simulink model "BBBC"  (R2022b)
settings: Solver=VariableStepAuto  StartTime=0.0  StopTime=0.5  RelTol=1e-3
undefined symbols (not defined in the file): dct, dEv, Ev, sigbuilder_block
libraries: spsSeriesRLCBranchLib x5, spsMosfetLib x4, simulink x3, spsVoltageMeasurementLib x2, spsGroundLib x1, spsCurrentMeasurementLib x1, spsControlledVoltageSourceLib x1, spspowerguiLib x1
settings Model: Creator=Dopechuro  LastModifiedBy=Dopechuro

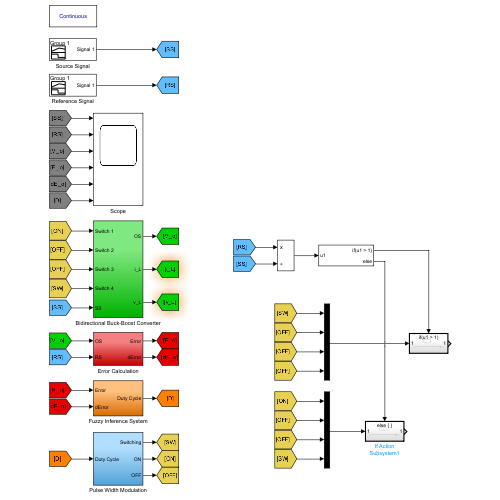
[thumbnail: Simulink's stored preview of the top-level diagram]
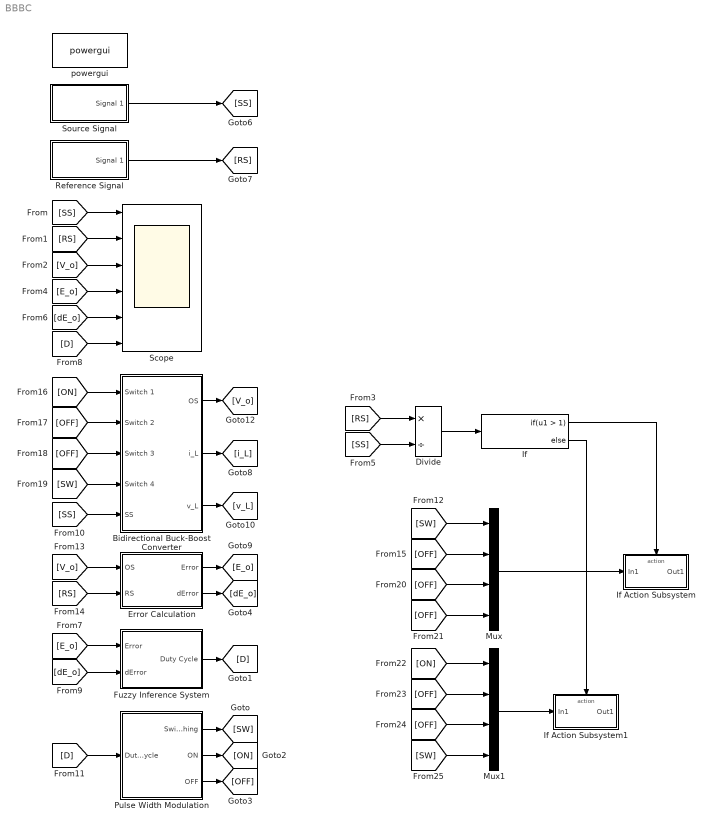
== system BBBC ==
  Bidirectional Buck-Boost Converter : Subsystem
  Divide : Product  Inputs=*/
  Error Calculation : Subsystem
  Fuzzy Inference System : Subsystem
  If : If  IfExpression=u1 > 1
  If Action Subsystem : Subsystem  TreatAsAtomicUnit=on
  If Action Subsystem1 : Subsystem  TreatAsAtomicUnit=on
  Mux : Mux
  Mux1 : Mux
  Pulse Width Modulation : Subsystem
  Reference Signal : Subsystem  Tag=STV Subsys  LoadFcn=sigbuilder_block('load');  StartFcn=sigbuilder_block('start');  StopFcn=sigbuilder_block('stop');  ClipboardFcn=sigbuilder_block('clipboard');  mask(Sigbuilder block){tuvar=[0:10]}
      mask help: Simulink:masks:SigbuilderBlock_MD
      mask init:
      | if ~strcmp(get_param(bdroot(gcbh),'SimulationStatus'),'stopped') tuvar = sigbuilder_block('maskInit'); end
      settings: CopyFcn=sigbuilder_block('copy');  DeleteFcn=sigbuilder_block('delete');  ModelCloseFcn=sigbuilder_block('modelClose');  PreSaveFcn=sigbuilder_block('preSave');  PauseFcn=sigbuilder_block('pause');  ContinueFcn=sigbuilder_block('continue');  NameChangeFcn=sigbuilder_block('namechange');  OpenFcn=sigbuilder_block('open',[530.25 309.75 550.5 399.75 ]);  CloseFcn=sigbuilder_block('close');
      mask Display: plot(0, 0, 100, 100,[2, 2, 32, 32, 2], [68, 8, 8, 68, 68],[32, 2], [38, 38], [32, 19, 2],[53, 60, 44], [32, 17, 17, 2],[16, 16, 31, 31]);txt = getActiveGroup(gcbh);text(2, 100, txt,'verticalAlignment', 'top');
  Scope : Scope  NumInputPorts=6
  Source Signal : Subsystem  Tag=STV Subsys  LoadFcn=sigbuilder_block('load');  StartFcn=sigbuilder_block('start');  StopFcn=sigbuilder_block('stop');  ClipboardFcn=sigbuilder_block('clipboard');  mask(Sigbuilder block){tuvar=[0:10]}
      mask help: Simulink:masks:SigbuilderBlock_MD
      mask init:
      | if ~strcmp(get_param(bdroot(gcbh),'SimulationStatus'),'stopped') tuvar = sigbuilder_block('maskInit'); end
      settings: CopyFcn=sigbuilder_block('copy');  DeleteFcn=sigbuilder_block('delete');  ModelCloseFcn=sigbuilder_block('modelClose');  PreSaveFcn=sigbuilder_block('preSave');  PauseFcn=sigbuilder_block('pause');  ContinueFcn=sigbuilder_block('continue');  NameChangeFcn=sigbuilder_block('namechange');  OpenFcn=sigbuilder_block('open',[395.25 256.5 550.5 399.75 ]);  CloseFcn=sigbuilder_block('close');
      mask Display: plot(0, 0, 100, 100,[2, 2, 32, 32, 2], [68, 8, 8, 68, 68],[32, 2], [38, 38], [32, 19, 2],[53, 60, 44], [32, 17, 17, 2],[16, 16, 31, 31]);txt = getActiveGroup(gcbh);text(2, 100, txt,'verticalAlignment', 'top');
  powergui : spspowerguiLib/powergui  Priority=1  SimulationMode=Continuous  SampleTime=50e-6  frequency=60  Iterations=50  frequencyindice=0  Pbase=100e6  ErrMax=1e-4  UnitsV=kV  UnitsW=MW  buscounter=0  FunctionMessages=off  echomessages=off  EnableUseOfTLC=off  CurrentSourceSwitches=off  DisableSnubberDevices=off  DisableRonSwitches=off  DisableVfSwitches=off  DisplayEquations=off  AutomaticDiscreteSolvers=off  SolverType=Tustin/Backward Euler (TBE)  Interpol=off  ExternalGateDelay=off  methode=off  Ts=100  x0status=blocks  SPID=on  SwTol=0  HookPort=off  NonlinearTolerance=1e-4  nMaxIteration=100  ContinueOnMaxIteration=off  RestoreLinks=warning  ResistiveCurrentMeasurement=off  Frange=[0:2:500]  Ylog=off  Xlog=on  ShowGrid=off  save=off  variable=ZData  structure=0  ZoomFFT=off  StartTime=0.0  cycles=1  DisplayStyle=1  fundamental=60  FreqAxis=off  MaxFrequency=1000  frequencyindicesteady=1  RmsSteady=1  display=off
  wires:
  [RS] -> Scope/2
  [V_o] -> Scope/3
  [E_o] -> Scope/4
  [dE_o] -> Scope/5
  [D] -> Scope/6
  Source Signal/1(Signal 1) -> [SS]
  Reference Signal/1(Signal 1) -> [RS]
  [V_o] -> Error Calculation/1(OS)
  [RS] -> Error Calculation/2(RS)
  Error Calculation/1(Error) -> [E_o]
  Error Calculation/2(dError) -> [dE_o]
  [SS] -> Scope/1
  [ON] -> Bidirectional Buck-Boost Converter/1(Switch 1)
  [OFF] -> Bidirectional Buck-Boost Converter/2(Switch 2)
  [OFF] -> Bidirectional Buck-Boost Converter/3(Switch 3)
  [SW] -> Bidirectional Buck-Boost Converter/4(Switch 4)
  [SS] -> Bidirectional Buck-Boost Converter/5(SS)
  Bidirectional Buck-Boost Converter/1(OS) -> [V_o]
  Bidirectional Buck-Boost Converter/2(i_L) -> [i_L]
  Bidirectional Buck-Boost Converter/3(v_L) -> [v_L]
  [E_o] -> Fuzzy Inference System/1(Error)
  [dE_o] -> Fuzzy Inference System/2(dError)
  Fuzzy Inference System/1(Duty Cycle) -> [D]
  [D] -> Pulse Width Modulation/1(Duty Cycle)
  Pulse Width Modulation/1(Switching) -> [SW]
  Pulse Width Modulation/2(ON) -> [ON]
  Pulse Width Modulation/3(OFF) -> [OFF]
  [SS] -> Divide/2
  [RS] -> Divide/1
  [SW] -> Mux/1
  [OFF] -> Mux/2
  [OFF] -> Mux/3
  [OFF] -> Mux/4
  [ON] -> Mux1/1
  [OFF] -> Mux1/2
  [OFF] -> Mux1/3
  [SW] -> Mux1/4
  Divide/1 -> If/1
  If/1 -> If Action Subsystem/Action
  If/2 -> If Action Subsystem1/Action
  Mux1/1 -> If Action Subsystem1/1(In1)
  Mux/1 -> If Action Subsystem/1(In1)

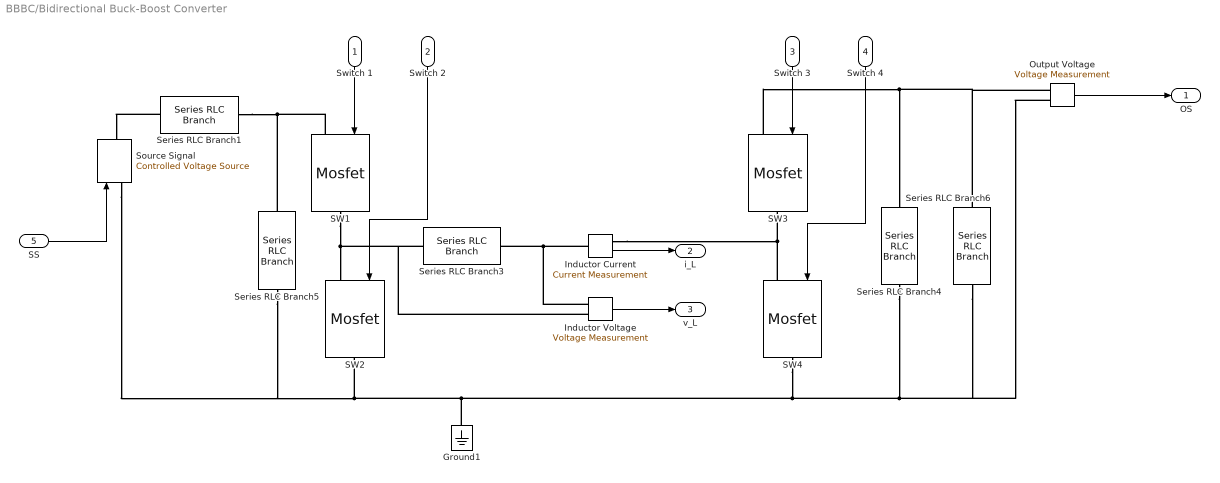
== system BBBC/Bidirectional Buck-Boost Converter ==
  Switch 1 : Inport
  Switch 2 : Inport  Port=2
  Switch 3 : Inport  Port=3
  Switch 4 : Inport  Port=4
  SS : Inport  Port=5
  Ground1 : spsGroundLib/Ground  LConnTagsString=a
  Inductor Current : spsCurrentMeasurementLib/Current Measurement  PhasorSimulation=off  OutputType=Complex  PSBequivalent=0
  Inductor Voltage : spsVoltageMeasurementLib/Voltage Measurement  PhasorSimulation=off  OutputType=Complex  PSBequivalent=0
  Output Voltage : spsVoltageMeasurementLib/Voltage Measurement  PhasorSimulation=off  OutputType=Complex  PSBequivalent=0
  SW{1..4} (4 alike) : spsMosfetLib/Mosfet  Ron=0.1  Lon=0  Rd=0.01  Vfd=0  IC=0  Rs=1e5  Cs=inf  Measurements=off
  Series RLC Branch1 : spsSeriesRLCBranchLib/Series RLC Branch  LConnTagsString=__new0  RConnTagsString=__new0  BranchType=R  Resistance=1e-6  Inductance=1e-3  SetiL0=off  InitialCurrent=0  Capacitance=1e-6  Setx0=off  InitialVoltage=0  Measurements=None
  Series RLC Branch3 : spsSeriesRLCBranchLib/Series RLC Branch  LConnTagsString=__new0  RConnTagsString=__new0  BranchType=L  Resistance=1  Inductance=22e-6  SetiL0=off  InitialCurrent=0  Capacitance=1e-6  Setx0=off  InitialVoltage=0  Measurements=None
  Series RLC Branch4 : spsSeriesRLCBranchLib/Series RLC Branch  LConnTagsString=__new0  RConnTagsString=__new0  BranchType=C  Resistance=1  Inductance=1e-3  SetiL0=off  InitialCurrent=0  Capacitance=1000e-6  Setx0=off  InitialVoltage=0  Measurements=None
  Series RLC Branch5 : spsSeriesRLCBranchLib/Series RLC Branch  LConnTagsString=__new0  RConnTagsString=__new0  BranchType=C  Resistance=1  Inductance=1e-3  SetiL0=off  InitialCurrent=0  Capacitance=1000e-6  Setx0=off  InitialVoltage=0  Measurements=None
  Series RLC Branch6 : spsSeriesRLCBranchLib/Series RLC Branch  LConnTagsString=__new0  RConnTagsString=__new0  BranchType=R  Resistance=5  Inductance=1e-3  SetiL0=off  InitialCurrent=0  Capacitance=1e-6  Setx0=off  InitialVoltage=0  Measurements=None
  Source Signal : spsControlledVoltageSourceLib/Controlled Voltage Source  Initialize=off  Source_Type=DC  Amplitude=0  Phase=0  Frequency=0  Measurements=None
  OS : Outport
  i_L : Outport  Port=2
  v_L : Outport  Port=3
  wires:
  Switch 1/1 -> SW1/1
  Switch 3/1 -> SW3/1
  Switch 2/1 -> SW2/1
  SS/1 -> Source Signal/1
  Switch 4/1 -> SW4/1
  Inductor Current/1 -> i_L/1
  Output Voltage/1 -> OS/1
  Inductor Voltage/1 -> v_L/1
  connections:
  Series RLC Branch5/LConn1 -- Series RLC Branch1/RConn1 -- SW1/LConn1
  Inductor Current/LConn1 -- Inductor Voltage/LConn2 -- Series RLC Branch3/RConn1
  SW4/LConn1 -- Inductor Current/RConn1 -- SW3/RConn1
  SW4/RConn1 -- Series RLC Branch6/RConn1 -- Output Voltage/LConn2 -- Series RLC Branch4/RConn1 -- Ground1/LConn1 -- Source Signal/LConn1 -- Series RLC Branch5/RConn1 -- SW2/RConn1
  SW1/RConn1 -- Inductor Voltage/LConn1 -- Series RLC Branch3/LConn1 -- SW2/LConn1
  Series RLC Branch1/LConn1 -- Source Signal/RConn1
  SW3/LConn1 -- Output Voltage/LConn1 -- Series RLC Branch6/LConn1 -- Series RLC Branch4/LConn1

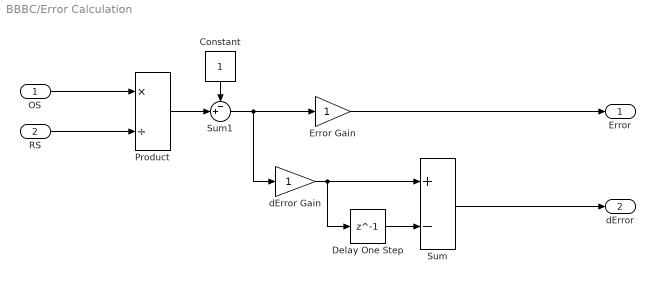
== system BBBC/Error Calculation ==
  OS : Inport
  RS : Inport  Port=2
  Constant : Constant
  Delay One Step : Delay  DelayLength=1
  Error Gain : Gain
  Product : Product  Inputs=*/
  Sum : Sum  Inputs=+-
  Sum1 : Sum  Inputs=-+|
  dError Gain : Gain
  Error : Outport
  dError : Outport  Port=2
  wires:
  Sum1/1 -> dError Gain/1, Error Gain/1
  dError Gain/1 -> Sum/1, Delay One Step/1
  Error Gain/1 -> Error/1
  Constant/1 -> Sum1/1
  Delay One Step/1 -> Sum/2
  Product/1 -> Sum1/2
  Sum/1 -> dError/1
  OS/1 -> Product/1
  RS/1 -> Product/2

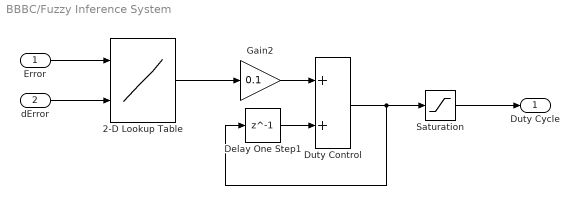
== system BBBC/Fuzzy Inference System ==
  Error : Inport
  dError : Inport  Port=2
  2-D Lookup Table : Lookup_n-D  LookupTableObject=''  BreakpointsForDimension1=Ev  BreakpointsForDimension2=dEv  BreakpointsForDimension1FirstPoint=10  BreakpointsForDimension2FirstPoint=10  BreakpointsForDimension1Spacing=12  BreakpointsForDimension2Spacing=12  IndexSearchMethod=Evenly spaced points  Table=dct  InterpMethod=Nearest  DiagnosticForOutOfRangeInput=Warning  InternalRulePriority=Speed  OutDataTypeStr=Inherit: Inherit from 'Table data'  RndMeth=Simplest
      settings: InputPortMap=u0,u1
  Delay One Step1 : Delay  DelayLength=1
  Duty Control : Sum
  Gain2 : Gain  Gain=0.1
  Saturation : Saturate  UpperLimit=0.4  LowerLimit=-0.4
  Duty Cycle : Outport
  wires:
  Delay One Step1/1 -> Duty Control/2
  Duty Control/1 -> Saturation/1, Delay One Step1/1
  Gain2/1 -> Duty Control/1
  2-D Lookup Table/1 -> Gain2/1
  Saturation/1 -> Duty Cycle/1
  Error/1 -> 2-D Lookup Table/1
  dError/1 -> 2-D Lookup Table/2

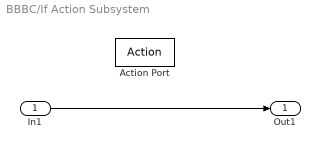
== system BBBC/If Action Subsystem ==
  In1 : Inport
  Action Port : ActionPort  ActionPortLabel=if(u1 > 1)
  Out1 : Outport
  wires:
  In1/1 -> Out1/1

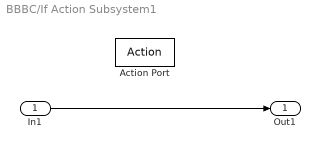
== system BBBC/If Action Subsystem1 ==
  In1 : Inport
  Action Port : ActionPort  ActionPortLabel=else
  Out1 : Outport
  wires:
  In1/1 -> Out1/1

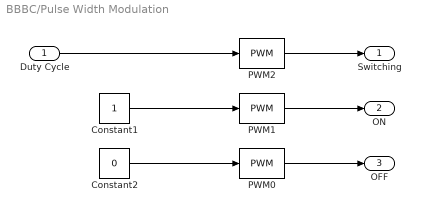
== system BBBC/Pulse Width Modulation ==
  Duty Cycle : Inport
  Constant1 : Constant
  Constant2 : Constant  Value=0
  PWM0 : simulink/Discontinuities/PWM  DisableCoverage=on  Period=1/1e4  InitialDelay=0  DisallowZeroDutyCycle=off  RunAtFixedTimeIntervals=off  SampleTime=0.1
  PWM1 : simulink/Discontinuities/PWM  DisableCoverage=on  Period=1/1e4  InitialDelay=0  DisallowZeroDutyCycle=off  RunAtFixedTimeIntervals=off  SampleTime=0.1
  PWM2 : simulink/Discontinuities/PWM  DisableCoverage=on  Period=1/1e4  InitialDelay=0  DisallowZeroDutyCycle=off  RunAtFixedTimeIntervals=off  SampleTime=0.1
  Switching : Outport
  ON : Outport  Port=2
  OFF : Outport  Port=3
  wires:
  Constant1/1 -> PWM1/1
  PWM0/1 -> OFF/1
  PWM2/1 -> Switching/1
  Constant2/1 -> PWM0/1
  Duty Cycle/1 -> PWM2/1
  PWM1/1 -> ON/1

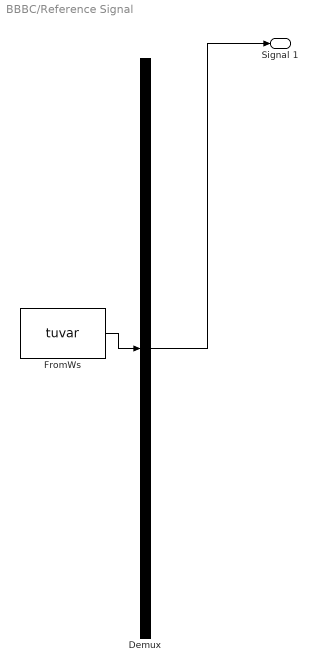
== system BBBC/Reference Signal ==
  Demux : Demux  Tag=STV Demux  Outputs=1
      settings: DisplayOption=none
  FromWs : FromWorkspace  Tag=STV FromWs  VariableName=tuvar
      SigBuilderData=|
      | common.afterFinalStr = 'Extrapolate'
      | common.sampleTime = 0
      | dataSet.timeRange = [0 1]
      | dataSet.name = 'Group 1'
      | sbobj.Groups.Name = 'Group 1'
      | sbobj.Groups.Signals.Name = 'Signal 1'
      | sbobj.Groups.Signals.XData = [0 1]
      | sbobj.Groups.Signals.YData = [3.3 3.3]
      | sbobj.Groups.TimeRange = [0 1]
  Signal 1 : Outport  Tag=STV Outport
  wires:
  FromWs/1 -> Demux/1
  Demux/1 -> Signal 1/1

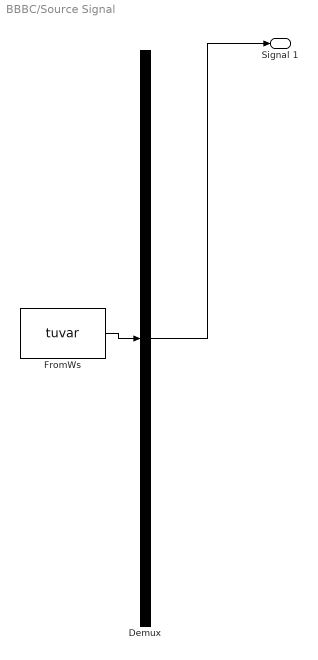
== system BBBC/Source Signal ==
  Demux : Demux  Tag=STV Demux  Outputs=1
      settings: DisplayOption=none
  FromWs : FromWorkspace  Tag=STV FromWs  VariableName=tuvar
      SigBuilderData=|
      | common.afterFinalStr = 'Extrapolate'
      | common.sampleTime = 0
      | dataSet.timeRange = [0 1]
      | dataSet.name = 'Group 1'
      | sbobj.Groups.Name = 'Group 1'
      | sbobj.Groups.Signals.Name = 'Signal 1'
      | sbobj.Groups.Signals.XData = [0 1]
      | sbobj.Groups.Signals.YData = [2.6 2.6]
      | sbobj.Groups.TimeRange = [0 1]
  Signal 1 : Outport  Tag=STV Outport
  wires:
  FromWs/1 -> Demux/1
  Demux/1 -> Signal 1/1
